simulink model "completofinal"  (Simulink 4.00)
settings: Solver=ode45  StartTime=0.0  StopTime=0.3  MaxStep=1/80000  RelTol=1e-3
libraries: simulink3 x2
settings Model: LastModifiedBy=Gui

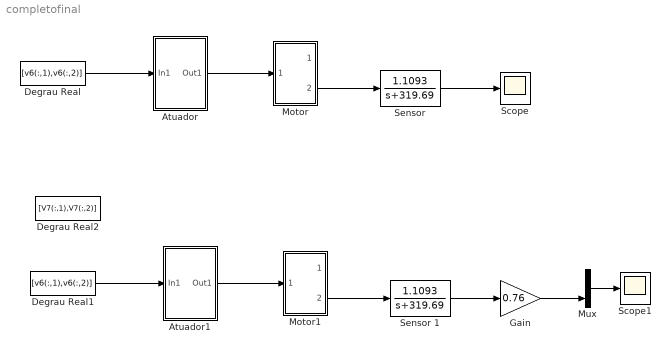
== system completofinal ==
  Atuador : Subsystem
      settings: RTWFcnNameOpts=Auto  RTWFileNameOpts=Auto
  Atuador1 : Subsystem
      settings: RTWFcnNameOpts=Auto  RTWFileNameOpts=Auto
  Degrau Real : FromWorkspace  VariableName=[v6(:,1),v6(:,2)]  SampleTime=0  OutputAfterFinalValue=Extrapolation
  Degrau Real1 : FromWorkspace  VariableName=[v6(:,1),v6(:,2)]  SampleTime=0  OutputAfterFinalValue=Extrapolation
  Degrau Real2 : FromWorkspace  VariableName=[V7(:,1),V7(:,2)]  SampleTime=0  OutputAfterFinalValue=Extrapolation
  Gain : Gain  Gain=0.76  Multiplication=Element-wise(K.*u)  SaturateOnIntegerOverflow=on
  Motor : Subsystem
      settings: RTWFcnNameOpts=Auto  RTWFileNameOpts=Auto
  Motor1 : Subsystem
      settings: RTWFcnNameOpts=Auto  RTWFileNameOpts=Auto
  Mux : Mux  Inputs=2
  Scope : Scope
      settings: TimeRange=0.06678048632136678  YMin=-0.486799  YMax=2.46879  SaveToWorkspace=off  SaveName=ScopeData  MaxDataPoints=5000
  Scope1 : Scope
      settings: TimeRange=0.06678048632136678  YMin=-0.486799  YMax=2.46879  SaveToWorkspace=off  SaveName=ScopeData2  MaxDataPoints=5000
  "Sensor " : TransferFcn  Numerator=1.1093  Denominator=[1 319.69]  AbsoluteTolerance=auto  Realization=auto
  Sensor 1 : TransferFcn  Numerator=1.1093  Denominator=[1 319.69]  AbsoluteTolerance=auto  Realization=auto
  wires:
  Atuador/1(Out1) -> Motor/1(In1)
  Motor/2(Out2) -> "Sensor "/1
  Degrau Real/1 -> Atuador/1(In1)
  "Sensor "/1 -> Scope/1
  Atuador1/1(Out1) -> Motor1/1(In1)
  Motor1/2(Out2) -> Sensor 1/1
  Degrau Real1/1 -> Atuador1/1(In1)
  Mux/1 -> Scope1/1
  Sensor 1/1 -> Gain/1
  Gain/1 -> Mux/2

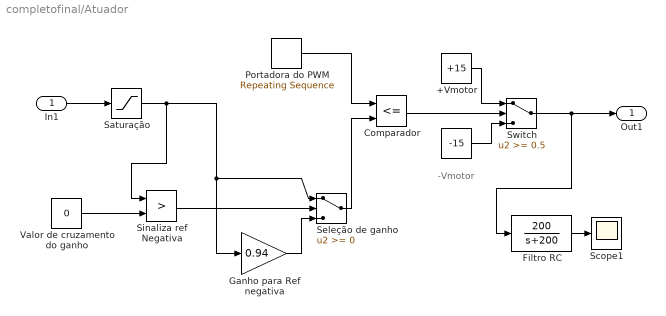
== system completofinal/Atuador ==
  note: -Vmotor
  In1 : Inport  Port=1  LatchInput=off
  " " : Constant  Value=-15
  +Vmotor : Constant  Value=+15
  Comparador : RelationalOperator  Operator=<=
  Filtro RC : TransferFcn  Numerator=[200]  Denominator=[1 200]  AbsoluteTolerance=auto  Realization=auto
  Ganho para Ref negativa : Gain  Gain=0.94  Multiplication=Element-wise(K.*u)  SaturateOnIntegerOverflow=on
  Portadora do PWM : simulink3/Sources/Repeating Sequence  rep_seq_t=[0 1/40000 1/20000]  rep_seq_y=[-10 10 -10]
  Saturação : Saturate  UpperLimit=9  LowerLimit=-10  LinearizeAsGain=on
  Scope1 : Scope
      settings: TimeRange=0.06  YMin=-14.11  YMax=-13.97  SaveToWorkspace=off  MaxDataPoints=5000
  Seleção de ganho : Switch  Threshold=0
  Sinaliza ref Negativa : RelationalOperator  Operator=>
  Switch : Switch  Threshold=0.5
  Valor de cruzamento do ganho : Constant  Value=0
  Out1 : Outport  Port=1
  wires:
  Comparador/1 -> Switch/2
  +Vmotor/1 -> Switch/1
  " "/1 -> Switch/3
  Portadora do PWM/1 -> Comparador/1
  In1/1 -> Saturação/1
  Switch/1 -> Filtro RC/1, Out1/1
  Seleção de ganho/1 -> Comparador/2
  Sinaliza ref Negativa/1 -> Seleção de ganho/2
  Valor de cruzamento do ganho/1 -> Sinaliza ref Negativa/2
  Saturação/1 -> Sinaliza ref Negativa/1, Ganho para Ref negativa/1, Seleção de ganho/1
  Ganho para Ref negativa/1 -> Seleção de ganho/3
  Filtro RC/1 -> Scope1/1

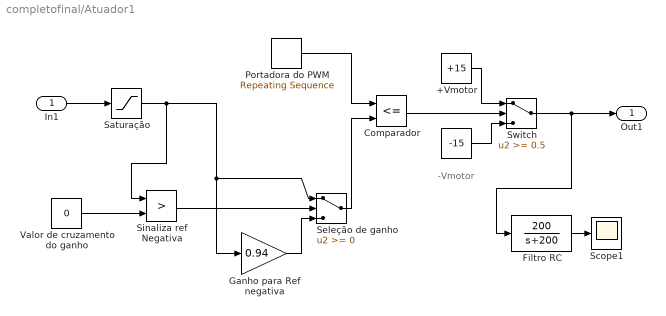
== system completofinal/Atuador1 ==
  note: -Vmotor
  In1 : Inport  Port=1  LatchInput=off
  " " : Constant  Value=-15
  +Vmotor : Constant  Value=+15
  Comparador : RelationalOperator  Operator=<=
  Filtro RC : TransferFcn  Numerator=[200]  Denominator=[1 200]  AbsoluteTolerance=auto  Realization=auto
  Ganho para Ref negativa : Gain  Gain=0.94  Multiplication=Element-wise(K.*u)  SaturateOnIntegerOverflow=on
  Portadora do PWM : simulink3/Sources/Repeating Sequence  rep_seq_t=[0 1/40000 1/20000]  rep_seq_y=[-10 10 -10]
  Saturação : Saturate  UpperLimit=9  LowerLimit=-10  LinearizeAsGain=on
  Scope1 : Scope
      settings: TimeRange=0.06  YMin=-14.11  YMax=-13.97  SaveToWorkspace=off  MaxDataPoints=5000
  Seleção de ganho : Switch  Threshold=0
  Sinaliza ref Negativa : RelationalOperator  Operator=>
  Switch : Switch  Threshold=0.5
  Valor de cruzamento do ganho : Constant  Value=0
  Out1 : Outport  Port=1
  wires:
  Comparador/1 -> Switch/2
  +Vmotor/1 -> Switch/1
  " "/1 -> Switch/3
  Portadora do PWM/1 -> Comparador/1
  In1/1 -> Saturação/1
  Switch/1 -> Filtro RC/1, Out1/1
  Seleção de ganho/1 -> Comparador/2
  Sinaliza ref Negativa/1 -> Seleção de ganho/2
  Valor de cruzamento do ganho/1 -> Sinaliza ref Negativa/2
  Saturação/1 -> Sinaliza ref Negativa/1, Ganho para Ref negativa/1, Seleção de ganho/1
  Ganho para Ref negativa/1 -> Seleção de ganho/3
  Filtro RC/1 -> Scope1/1

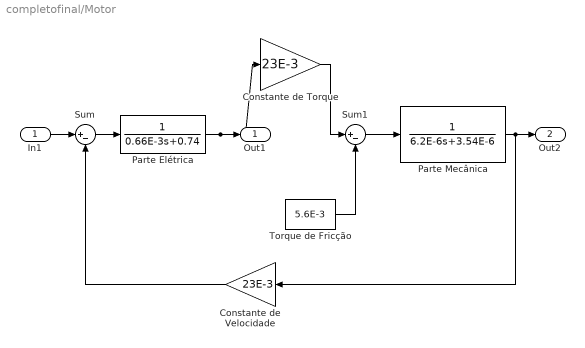
== system completofinal/Motor ==
  In1 : Inport  Port=1  LatchInput=off
  Constante de Torque : Gain  Gain=23E-3  Multiplication=Element-wise(K.*u)  SaturateOnIntegerOverflow=on
  Constante de Velocidade : Gain  Orientation=left  Gain=23E-3  Multiplication=Element-wise(K.*u)  SaturateOnIntegerOverflow=on
  Parte Elétrica : TransferFcn  Numerator=[1]  Denominator=[0.66E-3 0.74]  AbsoluteTolerance=auto  Realization=auto
  Parte Mecânica : TransferFcn  Numerator=[1]  Denominator=[6.2E-6 3.54E-6]  AbsoluteTolerance=auto  Realization=auto
  Sum : Sum  Inputs=|+-  SaturateOnIntegerOverflow=on
  Sum1 : Sum  Inputs=|+-  SaturateOnIntegerOverflow=on
  Torque de Fricção : Constant  Value=5.6E-3
  Out1 : Outport  Port=1
  Out2 : Outport  Port=2
  wires:
  Sum/1 -> Parte Elétrica/1
  Parte Elétrica/1 -> Constante de Torque/1, Out1/1
  Parte Mecânica/1 -> Constante de Velocidade/1, Out2/1
  Constante de Velocidade/1 -> Sum/2
  Constante de Torque/1 -> Sum1/1
  Sum1/1 -> Parte Mecânica/1
  Torque de Fricção/1 -> Sum1/2
  In1/1 -> Sum/1

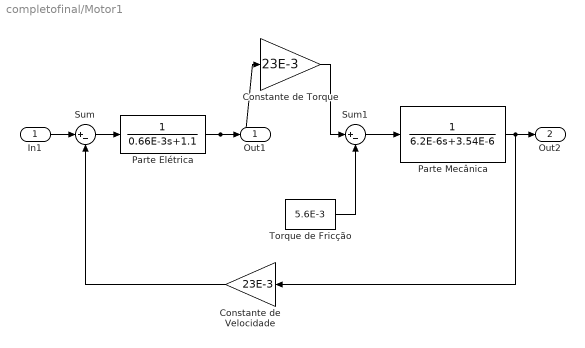
== system completofinal/Motor1 ==
  In1 : Inport  Port=1  LatchInput=off
  Constante de Torque : Gain  Gain=23E-3  Multiplication=Element-wise(K.*u)  SaturateOnIntegerOverflow=on
  Constante de Velocidade : Gain  Orientation=left  Gain=23E-3  Multiplication=Element-wise(K.*u)  SaturateOnIntegerOverflow=on
  Parte Elétrica : TransferFcn  Numerator=[1]  Denominator=[0.66E-3 1.1]  AbsoluteTolerance=auto  Realization=auto
  Parte Mecânica : TransferFcn  Numerator=[1]  Denominator=[6.2E-6 3.54E-6]  AbsoluteTolerance=auto  Realization=auto
  Sum : Sum  Inputs=|+-  SaturateOnIntegerOverflow=on
  Sum1 : Sum  Inputs=|+-  SaturateOnIntegerOverflow=on
  Torque de Fricção : Constant  Value=5.6E-3
  Out1 : Outport  Port=1
  Out2 : Outport  Port=2
  wires:
  Sum/1 -> Parte Elétrica/1
  Parte Elétrica/1 -> Constante de Torque/1, Out1/1
  Parte Mecânica/1 -> Constante de Velocidade/1, Out2/1
  Constante de Velocidade/1 -> Sum/2
  Constante de Torque/1 -> Sum1/1
  Sum1/1 -> Parte Mecânica/1
  Torque de Fricção/1 -> Sum1/2
  In1/1 -> Sum/1
